simulink model "exp2_latest_work_of_FULL_HEART_PICTURE_orignal_pure"  (R2023a)
settings: Solver=VariableStepAuto  StartTime=0.0  StopTime=60  RelTol=1e-3  AbsTol=1e-3
libraries: fl_lib x40, sh_lib x21, nesl_utility x18, simulink x7, Cardiovascular_lib x4
(part 1 of 2)
settings Model: Creator=luca  LastModifiedBy=Syed Abdul Rahman
settings SolverCC: AutoScaleAbsTol=off  ZeroCrossAlgorithm=Adaptive  AlgebraicLoopSolver=TrustRegion
settings DataIOCC: InspectSignalLogs=on
settings DebuggingCC: IgnoredZcDiagnostic=none  UnconnectedInputMsg=warning  UnconnectedOutputMsg=warning  UnconnectedLineMsg=warning  SymbolicDimsDataTypeCodeGenerationDiagnostic=none
settings ModelReferenceCC: EnableRefExpFcnMdlSchedulingChecks=on
settings SFSimCC: CustomCodeUndefinedFunction=UseInterfaceOnly
settings SimscapeCC: SimscapeLogType=all  SimscapeLogSimulationStatistics=on  SimscapeLogDataHistory=10000

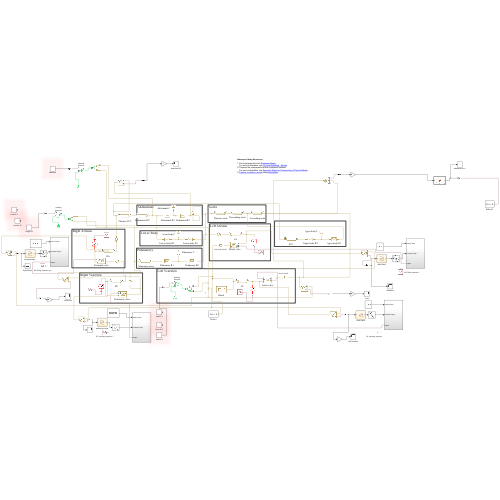
[thumbnail: Simulink's stored preview of the top-level diagram]
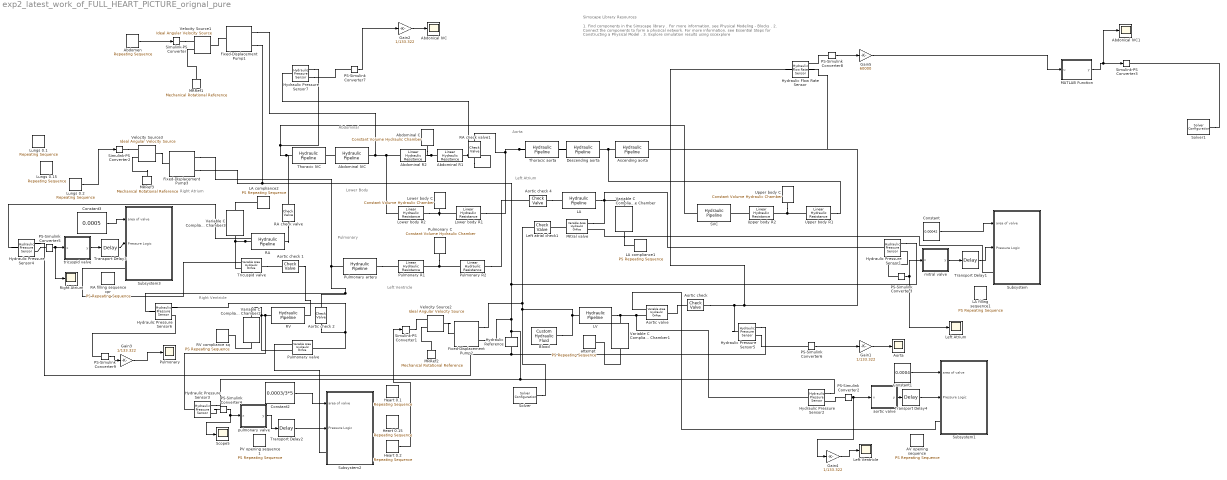
== system exp2_latest_work_of_FULL_HEART_PICTURE_orignal_pure ==
  note: Lower Body
  note: Left Atrium
  note: Right Ventricle
  note: Abdominal
  note: Aorta
  note: 1. Find components in the Simscape library .
      | For more information, see Physical Modeling - Blocks .
      | 2. Connect the components to form a physical network.
      | For more information, see Essential Steps for Constructing a Physical Model .
      | 3. Explore simulation results using sscexplore
  note: Simscape Library Resources
  note: Left Ventricle
  note: Right Atrium
  note: Pulmonary
  AV opening sequence : fl_lib/Physical Signals/Sources/PS Repeating Sequence  y_init=0  offset=0 s  sig_type=2  durations=[0.01 0.01 0.01 0.01 0.01 0.01 0.01 0.01 0.01 0.01 0.01 0.01 0.01 0.01 0.01 0.01 0.01 0.01 0.01 0.01 0.01 0.01 0.01 0.01 0.01 0.01 0.01 0.01 0.01 0.01 0.01 0.01 0.01 0.01 0.01 0.01 0.01 0.01 0.01 0.01 0.01 0.01 0.01 0.01 0.01 0.01 0.01 0.01 0.01 0.01 0.01 0.01 0.01 0.01 0.01 0.01 0.01 0.01 0.01 0.01 0.01 0.01 0.01 0.01 0.01 0.01 0.01 0.01 0.01 0.01 0.01 0.01 0.01 0.01 0.01 0.01 0.01 0.01 0.01 0.01 0.01 0.01 0.01 0.01 0.01 0.01 0.01 0.01 0.01 0.01 0.01 0.01 0.01 0.01 0.01 0.01 0.01 0.01 0.01 0.01] s  y_start="[0.000300000000000000\t0.000300000000000000\t0.000300000000000000\t0.000300000000000000\t0.000300000000000000\t0.000300000000000000\t0.000300000000000000\t0.000300000000000000\t0.000300000000000000\t0.000300000000000000\t0.000300000000000000\t0.000300000000000000\t0.000300000000000000\t0.000300000000000000\t0.000300000000000000\t0.000300000000000000\t0.000300000000000000\t0.000300000000000000\t0.000300000000000000\t0.000300000000000000\t0.000300000000000000\t0.000300000000000000\t0.000300000000000000\t0.000300000000000000\t0.000300000000000000\t0.000300000000000000\t0.000300000000000000\t0.000300000000000000\t0.000300000000000000\t0.000300000000000000\t0.000300000000000000\t0.000300000000000000\t0.000300000000000000\t0.000300000000000000\t0.000300000000000000\t0.000300000000000000\t0.000300000000000000\t0.000300000000000000\t0.000300000000000000\t0.000300000000000000\t0.000300000000000000\t0.000300000000000000\t0.000300000000000000\t0\t0\t0\t0\t0\t0\t0\t0\t0\t0\t0\t0\t0\t0\t0\t0\t0\t0\t0\t0\t0\t0\t0\t0\t0\t0\t0\t0\t0\t0\t0\t0\t0\t0\t0\t0\t0\t0\t0\t0\t0\t0\t0\t0\t0\t0\t0\t0\t0\t0\t0\t0\t0\t0\t0\t0\t0]/3*4"  y_end=1
      settings: InternalSimscapePortConfiguration="{\"Bottom\":[],\"Left\":[],\"Right\":[{\"id\":\"Y\",\"label\":\"Y\",\"type\":\"output\"}],\"Top\":[]}"
  "Abdomen " : simulink/Sources/Repeating Sequence  rep_seq_t=a1  rep_seq_y=a2
  Abdominal C : fl_lib/Hydraulic/Hydraulic Elements/Constant Volume Hydraulic Chamber  ch_sp=2  wall_type=2  ch_volume=1e-4 m^3  d_in=1 cm  length=2570.700637 cm  pr_r_coef=3.6E-08 m/Pa  time_const=0.01 s  k_sh=1.4  pressure_specify=off  pressure_priority=High  pressure=0 Pa  pressure_nominal_specify=off  pressure_nominal_unit=Pa  pressure_nominal_value=1  diameter_incr_specify=off  diameter_incr_priority=High  diameter_incr=0 m  diameter_incr_nominal_specify=off  diameter_incr_nominal_unit=m  diameter_incr_nominal_value=1  flow_rate_specify=off  flow_rate_priority=None  flow_rate=0.001 m^3/s  flow_rate_nominal_specify=off  flow_rate_nominal_unit=m^3/s  flow_rate_nominal_value=1
      settings: InternalSimscapePortConfiguration="{\"Bottom\":[],\"Left\":[{\"id\":\"A\",\"label\":\"\",\"type\":\"foundation.hydraulic.hydraulic\"}],\"Right\":[],\"Top\":[]}"
  Abdominal IVC : sh_lib/Pipelines/Hydraulic Pipeline  cs_type=1  d_in=1.37 cm  area=1e-4 m^2  D_h=1.12e-2 m  s_factor=64  length=17 cm  length_ad=0 m  roughness=15e-6 m  Re_lam=2000  Re_turb=4000  wall_type=2  pr_r_coef=4.39e-6 m/Pa  time_const=0.01 s  k_sh=1.4  initial_pressure=0 Pa
      settings: InternalSimscapePortConfiguration="{\"Bottom\":[],\"Left\":[{\"id\":\"A\",\"label\":\"A\",\"type\":\"foundation.hydraulic.hydraulic\"}],\"Right\":[{\"id\":\"B\",\"label\":\"B\",\"type\":\"foundation.hydraulic.hydraulic\"}],\"Top\":[]}"
  Abdominal R1 : fl_lib/Hydraulic/Hydraulic Elements/Linear Hydraulic Resistance  resistance=2.3e8 Pa/(m^3/s)  q_specify=off  q_priority=None  q=0.001 m^3/s  q_nominal_specify=off  q_nominal_unit=m^3/s  q_nominal_value=1  p_specify=off  p_priority=None  p=0 Pa  p_nominal_specify=off  p_nominal_unit=Pa  p_nominal_value=1
      settings: InternalSimscapePortConfiguration="{\"Bottom\":[],\"Left\":[{\"id\":\"A\",\"label\":\"A\",\"type\":\"foundation.hydraulic.hydraulic\"}],\"Right\":[{\"id\":\"B\",\"label\":\"B\",\"type\":\"foundation.hydraulic.hydraulic\"}],\"Top\":[]}"
  Abdominal R2 : fl_lib/Hydraulic/Hydraulic Elements/Linear Hydraulic Resistance  resistance=0.15e8 Pa/(m^3/s)  q_specify=off  q_priority=None  q=0.001 m^3/s  q_nominal_specify=off  q_nominal_unit=m^3/s  q_nominal_value=1  p_specify=off  p_priority=None  p=0 Pa  p_nominal_specify=off  p_nominal_unit=Pa  p_nominal_value=1
      settings: InternalSimscapePortConfiguration="{\"Bottom\":[],\"Left\":[{\"id\":\"A\",\"label\":\"A\",\"type\":\"foundation.hydraulic.hydraulic\"}],\"Right\":[{\"id\":\"B\",\"label\":\"B\",\"type\":\"foundation.hydraulic.hydraulic\"}],\"Top\":[]}"
  Abdonical IVC : Scope
  Abdonical IVC1 : Scope
  Aorta : Scope
  "Aortic check " : sh_lib/Valves/Directional Valves/Check Valve  area_max=1e-1 m^2  pres_crack=0.01 Pa  pres_max=0.1 Pa  C_d=1  A_leak=1e-12 m^2  lam_spec=1  B_lam=0.999  Re_cr=12  dynamic=0  tau=0.1 s  area_init=1e-12 m^2
      settings: InternalSimscapePortConfiguration="{\"Bottom\":[],\"Left\":[{\"id\":\"A\",\"label\":\"A\",\"type\":\"foundation.hydraulic.hydraulic\"}],\"Right\":[{\"id\":\"B\",\"label\":\"B\",\"type\":\"foundation.hydraulic.hydraulic\"}],\"Top\":[]}"
  Aortic check 1 : sh_lib/Valves/Directional Valves/Check Valve  area_max=1e-1 m^2  pres_crack=0.01 Pa  pres_max=0.1 Pa  C_d=1  A_leak=1e-12 m^2  lam_spec=1  B_lam=0.999  Re_cr=12  dynamic=0  tau=0.1 s  area_init=1e-12 m^2
      settings: InternalSimscapePortConfiguration="{\"Bottom\":[],\"Left\":[{\"id\":\"A\",\"label\":\"A\",\"type\":\"foundation.hydraulic.hydraulic\"}],\"Right\":[{\"id\":\"B\",\"label\":\"B\",\"type\":\"foundation.hydraulic.hydraulic\"}],\"Top\":[]}"
  Aortic check 2 : sh_lib/Valves/Directional Valves/Check Valve  area_max=1e-1 m^2  pres_crack=0.01 Pa  pres_max=0.1 Pa  C_d=1  A_leak=1e-12 m^2  lam_spec=1  B_lam=0.999  Re_cr=12  dynamic=0  tau=0.1 s  area_init=1e-12 m^2
      settings: InternalSimscapePortConfiguration="{\"Bottom\":[],\"Left\":[{\"id\":\"A\",\"label\":\"A\",\"type\":\"foundation.hydraulic.hydraulic\"}],\"Right\":[{\"id\":\"B\",\"label\":\"B\",\"type\":\"foundation.hydraulic.hydraulic\"}],\"Top\":[]}"
  Aortic check 4 : sh_lib/Valves/Directional Valves/Check Valve  area_max=1e-3 m^2  pres_crack=0.01 Pa  pres_max=0.1 Pa  C_d=1  A_leak=1e-12 m^2  lam_spec=1  B_lam=0.999  Re_cr=12  dynamic=0  tau=0.1 s  area_init=1e-12 m^2
      settings: InternalSimscapePortConfiguration="{\"Bottom\":[],\"Left\":[{\"id\":\"A\",\"label\":\"A\",\"type\":\"foundation.hydraulic.hydraulic\"}],\"Right\":[{\"id\":\"B\",\"label\":\"B\",\"type\":\"foundation.hydraulic.hydraulic\"}],\"Top\":[]}"
  Aortic valve : fl_lib/Hydraulic/Hydraulic Elements/Variable Area Hydraulic Orifice  C_d=1  min_area=1e-15 m^2  lam_spec=1  B_lam=0.999  Re_cr=12  q_specify=off  q_priority=None  q=0.001 m^3/s  q_nominal_specify=off  q_nominal_unit=m^3/s  q_nominal_value=1  p_specify=off  p_priority=None  p=0 Pa  p_nominal_specify=off  p_nominal_unit=Pa  p_nominal_value=1
      settings: InternalSimscapePortConfiguration="{\"Bottom\":[],\"Left\":[{\"id\":\"AR\",\"label\":\"AR\",\"type\":\"input\"},{\"id\":\"A\",\"label\":\"A\",\"type\":\"foundation.hydraulic.hydraulic\"}],\"Right\":[{\"id\":\"B\",\"label\":\"B\",\"type\":\"foundation.hydraulic.hydraulic\"}],\"Top\":[]}"
  Ascending aorta : sh_lib/Pipelines/Hydraulic Pipeline  cs_type=1  d_in=2.65 cm  area=1e-4 m^2  D_h=1.12e-2 m  s_factor=64  length=8.8 cm  length_ad=0 m  roughness=15e-6 m  Re_lam=2000  Re_turb=4000  wall_type=2  pr_r_coef=4.5e-7 m/Pa  time_const=0.01 s  k_sh=1.4  initial_pressure=0 Pa
      settings: InternalSimscapePortConfiguration="{\"Bottom\":[],\"Left\":[{\"id\":\"A\",\"label\":\"A\",\"type\":\"foundation.hydraulic.hydraulic\"}],\"Right\":[{\"id\":\"B\",\"label\":\"B\",\"type\":\"foundation.hydraulic.hydraulic\"}],\"Top\":[]}"
  "Blood " : fl_lib/Hydraulic/Hydraulic Utilities/Custom Hydraulic Fluid  density=1060 kg/m^3  viscosity_kin=3.55e-6 m^2/s  bulk=2.2e9 Pa  alpha=0.005  range_error=2
      settings: InternalSimscapePortConfiguration="{\"Bottom\":[],\"Left\":[],\"Right\":[{\"id\":\"G\",\"label\":\"\",\"type\":\"foundation.hydraulic.hydraulic\"}],\"Top\":[]}"
  Constant : Constant  Value=0.00042
  Constant1 : Constant  Value=0.0004
  Constant2 : Constant  Value=0.0003/3*5
  Constant3 : Constant  Value=0.0005
  Descending aorta : sh_lib/Pipelines/Hydraulic Pipeline  cs_type=1  d_in=2.15 cm  area=1e-4 m^2  D_h=1.12e-2 m  s_factor=64  length=6.94 cm  length_ad=0 m  roughness=15e-6 m  Re_lam=2000  Re_turb=4000  wall_type=2  pr_r_coef=1.4e-6 m/Pa  time_const=0.01 s  k_sh=1.4  initial_pressure=0 Pa
      settings: InternalSimscapePortConfiguration="{\"Bottom\":[],\"Left\":[{\"id\":\"A\",\"label\":\"A\",\"type\":\"foundation.hydraulic.hydraulic\"}],\"Right\":[{\"id\":\"B\",\"label\":\"B\",\"type\":\"foundation.hydraulic.hydraulic\"}],\"Top\":[]}"
  Fixed-Displacement Pump1 : sh_lib/Pumps and Motors/Fixed-Displacement Pump  D=13.33 cm^3/rev  loss_spec=1  w_nominal=20 rpm  pr_nominal=100e5 Pa  visc_nominal=3.55e-6 m^2/s  dens_nominal=1060 kg/m^3  efficiency_vol=0.92  no_load_torque=0.05 N*m  torque_pressure_coeff=0.6e-6 N*m/Pa  p_diff_eff_TLU=[100000, 1000000, 2000000] Pa  omega_eff_TLU=[25, 50, 100, 200, 300, 400] rad/s  vol_eff_TLU=[.816, .908, .954, .977, .981, .984; .325, .663, .831, .916, .925, .946; .137, .568, .78, .892, .893, .91]  mech_eff_TLU=[.996, .996, .996, .996, .996, .996; .988, .989, .989, .989, .989, .99; .981, .981, .982, .982, .983, .984]  p_diff_loss_TLU=[100000, 1000000, 2000000] Pa  omega_loss_TLU=[25, 50, 100, 200, 300, 400] rad/s  vol_loss_TLU=[.023, .023, .023, .023, .0285, .032; .0844, .0842, .0845, .084, .1125, .108; .1079, .108, .11, .108, .1605, .18] * 1e-3 m^3/s  mech_loss_TLU=[.002, .002, .002, .002, .002, .002; .0607, .0556, .0556, .0556, .0556, .0505; .1937, .1937, .1833, .1833, .1729, .1626] N*m  pressure_threshold=1e5 Pa  omega_threshold=10 rad/s  quadrant_check=0  pressure_check=0  min_valid_pressure=0 Pa  vol_eff_min=1e-3  vol_eff_max=1  mech_eff_min=1e-3  mech_eff_max=1
      settings: InternalSimscapePortConfiguration="{\"Bottom\":[],\"Left\":[{\"id\":\"S\",\"label\":\"S\",\"type\":\"foundation.mechanical.rotational.rotational\"}],\"Right\":[{\"id\":\"P\",\"label\":\"P\",\"type\":\"foundation.hydraulic.hydraulic\"},{\"id\":\"T\",\"label\":\"T\",\"type\":\"foundation.hydraulic.hydraulic\"}],\"Top\":[]}"
  Fixed-Displacement Pump2 : sh_lib/Pumps and Motors/Fixed-Displacement Pump  D=13.33 cm^3/rev  loss_spec=1  w_nominal=20 rpm  pr_nominal=100e5 Pa  visc_nominal=3.55e-6 m^2/s  dens_nominal=1060 kg/m^3  efficiency_vol=0.92  no_load_torque=0.05 N*m  torque_pressure_coeff=0.6e-6 N*m/Pa  p_diff_eff_TLU=[100000, 1000000, 2000000] Pa  omega_eff_TLU=[25, 50, 100, 200, 300, 400] rad/s  vol_eff_TLU=[.816, .908, .954, .977, .981, .984; .325, .663, .831, .916, .925, .946; .137, .568, .78, .892, .893, .91]  mech_eff_TLU=[.996, .996, .996, .996, .996, .996; .988, .989, .989, .989, .989, .99; .981, .981, .982, .982, .983, .984]  p_diff_loss_TLU=[100000, 1000000, 2000000] Pa  omega_loss_TLU=[25, 50, 100, 200, 300, 400] rad/s  vol_loss_TLU=[.023, .023, .023, .023, .0285, .032; .0844, .0842, .0845, .084, .1125, .108; .1079, .108, .11, .108, .1605, .18] * 1e-3 m^3/s  mech_loss_TLU=[.002, .002, .002, .002, .002, .002; .0607, .0556, .0556, .0556, .0556, .0505; .1937, .1937, .1833, .1833, .1729, .1626] N*m  pressure_threshold=1e5 Pa  omega_threshold=10 rad/s  quadrant_check=0  pressure_check=0  min_valid_pressure=0 Pa  vol_eff_min=1e-3  vol_eff_max=1  mech_eff_min=1e-3  mech_eff_max=1
      settings: InternalSimscapePortConfiguration="{\"Bottom\":[],\"Left\":[{\"id\":\"S\",\"label\":\"S\",\"type\":\"foundation.mechanical.rotational.rotational\"}],\"Right\":[{\"id\":\"P\",\"label\":\"P\",\"type\":\"foundation.hydraulic.hydraulic\"},{\"id\":\"T\",\"label\":\"T\",\"type\":\"foundation.hydraulic.hydraulic\"}],\"Top\":[]}"
  Fixed-Displacement Pump3 : sh_lib/Pumps and Motors/Fixed-Displacement Pump  D=13.33 cm^3/rev  loss_spec=1  w_nominal=20 rpm  pr_nominal=100e5 Pa  visc_nominal=3.55e-6 m^2/s  dens_nominal=1060 kg/m^3  efficiency_vol=0.92  no_load_torque=0.05 N*m  torque_pressure_coeff=0.6e-6 N*m/Pa  p_diff_eff_TLU=[100000, 1000000, 2000000] Pa  omega_eff_TLU=[25, 50, 100, 200, 300, 400] rad/s  vol_eff_TLU=[.816, .908, .954, .977, .981, .984; .325, .663, .831, .916, .925, .946; .137, .568, .78, .892, .893, .91]  mech_eff_TLU=[.996, .996, .996, .996, .996, .996; .988, .989, .989, .989, .989, .99; .981, .981, .982, .982, .983, .984]  p_diff_loss_TLU=[100000, 1000000, 2000000] Pa  omega_loss_TLU=[25, 50, 100, 200, 300, 400] rad/s  vol_loss_TLU=[.023, .023, .023, .023, .0285, .032; .0844, .0842, .0845, .084, .1125, .108; .1079, .108, .11, .108, .1605, .18] * 1e-3 m^3/s  mech_loss_TLU=[.002, .002, .002, .002, .002, .002; .0607, .0556, .0556, .0556, .0556, .0505; .1937, .1937, .1833, .1833, .1729, .1626] N*m  pressure_threshold=1e5 Pa  omega_threshold=10 rad/s  quadrant_check=0  pressure_check=0  min_valid_pressure=0 Pa  vol_eff_min=1e-3  vol_eff_max=1  mech_eff_min=1e-3  mech_eff_max=1
      settings: InternalSimscapePortConfiguration="{\"Bottom\":[],\"Left\":[{\"id\":\"S\",\"label\":\"S\",\"type\":\"foundation.mechanical.rotational.rotational\"}],\"Right\":[{\"id\":\"P\",\"label\":\"P\",\"type\":\"foundation.hydraulic.hydraulic\"},{\"id\":\"T\",\"label\":\"T\",\"type\":\"foundation.hydraulic.hydraulic\"}],\"Top\":[]}"
  Gain{1..4} (4 alike) : Gain  Gain=1/133.322
  Gain5 : Gain  Gain=60000
  Heart 0.1 : simulink/Sources/Repeating Sequence  rep_seq_t=b1  rep_seq_y=b2
  Heart 0.15 : simulink/Sources/Repeating Sequence  rep_seq_t=c1  rep_seq_y=c2
  Heart 0.2 : simulink/Sources/Repeating Sequence  rep_seq_t=d1  rep_seq_y=d2
  Hydraulic Flow Rate Sensor : fl_lib/Hydraulic/Hydraulic Sensors/Hydraulic Flow Rate Sensor
  Hydraulic Pressure Sensor{1..7} (7 alike) : fl_lib/Hydraulic/Hydraulic Sensors/Hydraulic Pressure Sensor
  Hydraulic Reference : fl_lib/Hydraulic/Hydraulic Elements/Hydraulic Reference
  LA : sh_lib/Pipelines/Hydraulic Pipeline  cs_type=1  d_in=4.8 cm  area=1e-4 m^2  D_h=1.12e-2 m  s_factor=64  length=5 cm  length_ad=0 m  roughness=15e-6 m  Re_lam=2000  Re_turb=4000  wall_type=1  pr_r_coef=5.9e-6 m/Pa  time_const=0.01 s  k_sh=1.4  initial_pressure=0 Pa
      settings: InternalSimscapePortConfiguration="{\"Bottom\":[],\"Left\":[{\"id\":\"A\",\"label\":\"A\",\"type\":\"foundation.hydraulic.hydraulic\"}],\"Right\":[{\"id\":\"B\",\"label\":\"B\",\"type\":\"foundation.hydraulic.hydraulic\"}],\"Top\":[]}"
  LA compliance1 : fl_lib/Physical Signals/Sources/PS Repeating Sequence  y_init=0  offset=0 s  sig_type=2  durations=[0.01 0.01 0.01 0.01 0.01 0.01 0.01 0.01 0.01 0.01 0.01 0.01 0.01 0.01 0.01 0.01 0.01 0.01 0.01 0.01 0.01 0.01 0.01 0.01 0.01 0.01 0.01 0.01 0.01 0.01 0.01 0.01 0.01 0.01 0.01 0.01 0.01 0.01 0.01 0.01 0.01 0.01 0.01 0.01 0.01 0.01 0.01 0.01 0.01 0.01 0.01 0.01 0.01 0.01 0.01 0.01 0.01 0.01 0.01 0.01 0.01 0.01 0.01 0.01 0.01 0.01 0.01 0.01 0.01 0.01 0.01 0.01 0.01 0.01 0.01 0.01 0.01 0.01 0.01 0.01 0.01 0.01 0.01 0.01 0.01 0.01 0.01 0.01 0.01 0.01 0.01 0.01 0.01 0.01 0.01 0.01 0.01 0.01 0.01 0.01] s  y_start="[1.36500000000000e-05\t1.36862500000000e-05\t1.37225000000000e-05\t1.37587500000000e-05\t1.37950000000000e-05\t1.38312500000000e-05\t1.38675000000000e-05\t1.39037500000000e-05\t1.39400000000000e-05\t1.39762500000000e-05\t1.40125000000000e-05\t1.40487500000000e-05\t1.40850000000000e-05\t1.41212500000000e-05\t1.41575000000000e-05\t1.41937500000000e-05\t1.42300000000000e-05\t1.42662500000000e-05\t1.43025000000000e-05\t1.43387500000000e-05\t1.43750000000000e-05\t1.44112500000000e-05\t1.44475000000000e-05\t1.44837500000000e-05\t1.45200000000000e-05\t1.45562500000000e-05\t1.45925000000000e-05\t1.46287500000000e-05\t1.46650000000000e-05\t1.47012500000000e-05\t1.47375000000000e-05\t1.47737500000000e-05\t1.48100000000000e-05\t1.48462500000000e-05\t1.48825000000000e-05\t1.49187500000000e-05\t1.49550000000000e-05\t1.49912500000000e-05\t1.50275000000000e-05\t1.50637500000000e-05\t1.51000000000000e-05\t1.51362500000000e-05\t1.51725000000000e-05\t1.52087500000000e-05\t1.52450000000000e-05\t1.52812500000000e-05\t1.53175000000000e-05\t1.53537500000000e-05\t1.53900000000000e-05\t1.54262500000000e-05\t1.54625000000000e-05\t1.54987500000000e-05\t1.55350000000000e-05\t1.55712500000000e-05\t1.56075000000000e-05\t1.56437500000000e-05\t1.56800000000000e-05\t1.57162500000000e-05\t1.57525000000000e-05\t1.57887500000000e-05\t1.58250000000000e-05\t1.58612500000000e-05\t1.58975000000000e-05\t1.59337500000000e-05\t1.59700000000000e-05\t1.60062500000000e-05\t1.60425000000000e-05\t1.60787500000000e-05\t1.61150000000000e-05\t1.61512500000000e-05\t1.61875000000000e-05\t1.62237500000000e-05\t1.62600000000000e-05\t1.62962500000000e-05\t1.63325000000000e-05\t1.63687500000000e-05\t1.64050000000000e-05\t1.64412500000000e-05\t1.64775000000000e-05\t1.65137500000000e-05\t1.36500000000000e-05\t1.29125270139567e-05\t1.21876723951708e-05\t1.14878386071372e-05\t1.08250000000000e-05\t1.02104979261007e-05\t9.65484668629601e-06\t9.16755362735452e-06\t8.75695646861792e-06\t8.43008064131123e-06\t8.19251908146676e-06\t8.04833653323797e-06\t8.00000000000000e-06\t8.14165729617270e-06\t8.55952589635133e-06\t9.23265212405563e-06\t1.01272826194982e-05\t1.11985568739858e-05\t1.23927567231468e-05\t1.36500000000000e-05]"  y_end=1
      settings: InternalSimscapePortConfiguration="{\"Bottom\":[],\"Left\":[],\"Right\":[{\"id\":\"Y\",\"label\":\"Y\",\"type\":\"output\"}],\"Top\":[]}"
  LA compliance2 : fl_lib/Physical Signals/Sources/PS Repeating Sequence  y_init=0  offset=0 s  sig_type=2  durations=[0.01 0.01 0.01 0.01 0.01 0.01 0.01 0.01 0.01 0.01 0.01 0.01 0.01 0.01 0.01 0.01 0.01 0.01 0.01 0.01 0.01 0.01 0.01 0.01 0.01 0.01 0.01 0.01 0.01 0.01 0.01 0.01 0.01 0.01 0.01 0.01 0.01 0.01 0.01 0.01 0.01 0.01 0.01 0.01 0.01 0.01 0.01 0.01 0.01 0.01 0.01 0.01 0.01 0.01 0.01 0.01 0.01 0.01 0.01 0.01 0.01 0.01 0.01 0.01 0.01 0.01 0.01 0.01 0.01 0.01 0.01 0.01 0.01 0.01 0.01 0.01 0.01 0.01 0.01 0.01 0.01 0.01 0.01 0.01 0.01 0.01 0.01 0.01 0.01 0.01 0.01 0.01 0.01 0.01 0.01 0.01 0.01 0.01 0.01 0.01] s  y_start="[2.18400000000000e-05\t2.18580000000000e-05\t2.18760000000000e-05\t2.18940000000000e-05\t2.19120000000000e-05\t2.19300000000000e-05\t2.19480000000000e-05\t2.19660000000000e-05\t2.19840000000000e-05\t2.20020000000000e-05\t2.20200000000000e-05\t2.20380000000000e-05\t2.20560000000000e-05\t2.20740000000000e-05\t2.20920000000000e-05\t2.21100000000000e-05\t2.21280000000000e-05\t2.21460000000000e-05\t2.21640000000000e-05\t2.21820000000000e-05\t2.22000000000000e-05\t2.22180000000000e-05\t2.22360000000000e-05\t2.22540000000000e-05\t2.22720000000000e-05\t2.22900000000000e-05\t2.23080000000000e-05\t2.23260000000000e-05\t2.23440000000000e-05\t2.23620000000000e-05\t2.23800000000000e-05\t2.23980000000000e-05\t2.24160000000000e-05\t2.24340000000000e-05\t2.24520000000000e-05\t2.24700000000000e-05\t2.24880000000000e-05\t2.25060000000000e-05\t2.25240000000000e-05\t2.25420000000000e-05\t2.25600000000000e-05\t2.25780000000000e-05\t2.25960000000000e-05\t2.26140000000000e-05\t2.26320000000000e-05\t2.26500000000000e-05\t2.26680000000000e-05\t2.26860000000000e-05\t2.27040000000000e-05\t2.27220000000000e-05\t2.27400000000000e-05\t2.27580000000000e-05\t2.27760000000000e-05\t2.27940000000000e-05\t2.28120000000000e-05\t2.28300000000000e-05\t2.28480000000000e-05\t2.28660000000000e-05\t2.28840000000000e-05\t2.29020000000000e-05\t2.29200000000000e-05\t2.29380000000000e-05\t2.29560000000000e-05\t2.29740000000000e-05\t2.29920000000000e-05\t2.30100000000000e-05\t2.30280000000000e-05\t2.30460000000000e-05\t2.30640000000000e-05\t2.30820000000000e-05\t2.31000000000000e-05\t2.31180000000000e-05\t2.31360000000000e-05\t2.31540000000000e-05\t2.31720000000000e-05\t2.31900000000000e-05\t2.32080000000000e-05\t2.32260000000000e-05\t2.32440000000000e-05\t2.32620000000000e-05\t2.18400000000000e-05\t2.14693056140951e-05\t2.11049539119088e-05\t2.07531790520831e-05\t2.04200000000000e-05\t2.01111175416152e-05\t1.98318167414302e-05\t1.95868765135729e-05\t1.93804878532522e-05\t1.92161821276679e-05\t1.90967706533390e-05\t1.90242965936984e-05\t1.90000000000000e-05\t1.90712047294036e-05\t1.92812484151571e-05\t1.96195985897908e-05\t2.00692889627212e-05\t2.06077701809061e-05\t2.12080405475641e-05\t2.18400000000000e-05]"  y_end=1
      settings: InternalSimscapePortConfiguration="{\"Bottom\":[],\"Left\":[],\"Right\":[{\"id\":\"Y\",\"label\":\"Y\",\"type\":\"output\"}],\"Top\":[]}"
  LA filling sequence1 : fl_lib/Physical Signals/Sources/PS Repeating Sequence  y_init=0  offset=0 s  sig_type=2  durations=[0.01 0.01 0.01 0.01 0.01 0.01 0.01 0.01 0.01 0.01 0.01 0.01 0.01 0.01 0.01 0.01 0.01 0.01 0.01 0.01 0.01 0.01 0.01 0.01 0.01 0.01 0.01 0.01 0.01 0.01 0.01 0.01 0.01 0.01 0.01 0.01 0.01 0.01 0.01 0.01 0.01 0.01 0.01 0.01 0.01 0.01 0.01 0.01 0.01 0.01 0.01 0.01 0.01 0.01 0.01 0.01 0.01 0.01 0.01 0.01 0.01 0.01 0.01 0.01 0.01 0.01 0.01 0.01 0.01 0.01 0.01 0.01 0.01 0.01 0.01 0.01 0.01 0.01 0.01 0.01 0.01 0.01 0.01 0.01 0.01 0.01 0.01 0.01 0.01 0.01 0.01 0.01 0.01 0.01 0.01 0.01 0.01 0.01 0.01 0.01] s  y_start="[0\t0\t0\t0\t0\t0\t0\t0\t0\t0\t0\t0\t0\t0\t0\t0\t0\t0\t0\t0\t0\t0\t0\t0\t0\t0\t0\t0\t0\t0\t0\t0\t0\t0\t0\t0\t0\t0\t0\t0\t0\t0\t0\t0\t0\t0.000420000000000000\t0.000420000000000000\t0.000420000000000000\t0.000420000000000000\t0.000420000000000000\t0.000420000000000000\t0.000420000000000000\t0.000420000000000000\t0.000420000000000000\t0.000420000000000000\t0.000420000000000000\t0.000420000000000000\t0.000420000000000000\t0.000420000000000000\t0.000420000000000000\t0.000420000000000000\t0.000420000000000000\t0.000420000000000000\t0.000420000000000000\t0.000420000000000000\t0.000420000000000000\t0.000420000000000000\t0.000420000000000000\t0.000420000000000000\t0.000420000000000000\t0.000420000000000000\t0.000420000000000000\t0.000420000000000000\t0.000420000000000000\t0.000420000000000000\t0.000420000000000000\t0.000420000000000000\t0.000420000000000000\t0.000420000000000000\t0.000420000000000000\t0.000420000000000000\t0.000420000000000000\t0.000420000000000000\t0.000420000000000000\t0.000420000000000000\t0.000420000000000000\t0.000420000000000000\t0.000420000000000000\t0.000420000000000000\t0.000420000000000000\t0.000420000000000000\t0.000420000000000000\t0.000420000000000000\t0.000420000000000000\t0.000420000000000000\t0.000420000000000000\t0.000420000000000000\t0.000420000000000000\t0.000420000000000000\t0.000420000000000000]"  y_end=1
      settings: InternalSimscapePortConfiguration="{\"Bottom\":[],\"Left\":[],\"Right\":[{\"id\":\"Y\",\"label\":\"Y\",\"type\":\"output\"}],\"Top\":[]}"
  LV : sh_lib/Pipelines/Hydraulic Pipeline  cs_type=1  d_in=4.4 cm  area=1e-4 m^2  D_h=1.12e-2 m  s_factor=64  length=7 cm  length_ad=0 m  roughness=15e-6 m  Re_lam=2000  Re_turb=4000  wall_type=1  pr_r_coef=3.8e-7 m/Pa  time_const=0.01 s  k_sh=1.4  initial_pressure=0 Pa
      settings: InternalSimscapePortConfiguration="{\"Bottom\":[],\"Left\":[{\"id\":\"A\",\"label\":\"A\",\"type\":\"foundation.hydraulic.hydraulic\"}],\"Right\":[{\"id\":\"B\",\"label\":\"B\",\"type\":\"foundation.hydraulic.hydraulic\"}],\"Top\":[]}"
  "Left Atrium " : Scope
  Left Ventricle : Scope
  Left atrial check1 : sh_lib/Valves/Directional Valves/Check Valve  area_max=1e-1 m^2  pres_crack=0.01 Pa  pres_max=0.1 Pa  C_d=0.7  A_leak=1e-12 m^2  lam_spec=1  B_lam=0.999  Re_cr=12  dynamic=0  tau=0.1 s  area_init=1e-12 m^2
      settings: InternalSimscapePortConfiguration="{\"Bottom\":[],\"Left\":[{\"id\":\"A\",\"label\":\"A\",\"type\":\"foundation.hydraulic.hydraulic\"}],\"Right\":[{\"id\":\"B\",\"label\":\"B\",\"type\":\"foundation.hydraulic.hydraulic\"}],\"Top\":[]}"
  Lower body C : fl_lib/Hydraulic/Hydraulic Elements/Constant Volume Hydraulic Chamber  ch_sp=2  wall_type=2  ch_volume=1e-4 m^3  d_in=1 cm  length=648.4076433 cm  pr_r_coef=4.1E-08 m/Pa  time_const=0.01 s  k_sh=1.4  pressure_specify=off  pressure_priority=High  pressure=0 Pa  pressure_nominal_specify=off  pressure_nominal_unit=Pa  pressure_nominal_value=1  diameter_incr_specify=off  diameter_incr_priority=High  diameter_incr=0 m  diameter_incr_nominal_specify=off  diameter_incr_nominal_unit=m  diameter_incr_nominal_value=1  flow_rate_specify=off  flow_rate_priority=None  flow_rate=0.001 m^3/s  flow_rate_nominal_specify=off  flow_rate_nominal_unit=m^3/s  flow_rate_nominal_value=1
      settings: InternalSimscapePortConfiguration="{\"Bottom\":[],\"Left\":[{\"id\":\"A\",\"label\":\"\",\"type\":\"foundation.hydraulic.hydraulic\"}],\"Right\":[],\"Top\":[]}"
  Lower body R1 : fl_lib/Hydraulic/Hydraulic Elements/Linear Hydraulic Resistance  resistance=4.79e8 Pa/(m^3/s)  q_specify=off  q_priority=None  q=0.001 m^3/s  q_nominal_specify=off  q_nominal_unit=m^3/s  q_nominal_value=1  p_specify=off  p_priority=None  p=0 Pa  p_nominal_specify=off  p_nominal_unit=Pa  p_nominal_value=1
      settings: InternalSimscapePortConfiguration="{\"Bottom\":[],\"Left\":[{\"id\":\"A\",\"label\":\"A\",\"type\":\"foundation.hydraulic.hydraulic\"}],\"Right\":[{\"id\":\"B\",\"label\":\"B\",\"type\":\"foundation.hydraulic.hydraulic\"}],\"Top\":[]}"
  Lower body R2 : fl_lib/Hydraulic/Hydraulic Elements/Linear Hydraulic Resistance  resistance=0.4e8 Pa/(m^3/s)  q_specify=off  q_priority=None  q=0.001 m^3/s  q_nominal_specify=off  q_nominal_unit=m^3/s  q_nominal_value=1  p_specify=off  p_priority=None  p=0 Pa  p_nominal_specify=off  p_nominal_unit=Pa  p_nominal_value=1
      settings: InternalSimscapePortConfiguration="{\"Bottom\":[],\"Left\":[{\"id\":\"A\",\"label\":\"A\",\"type\":\"foundation.hydraulic.hydraulic\"}],\"Right\":[{\"id\":\"B\",\"label\":\"B\",\"type\":\"foundation.hydraulic.hydraulic\"}],\"Top\":[]}"
  Lungs 0.1 : simulink/Sources/Repeating Sequence  rep_seq_t=m1  rep_seq_y=m2
  Lungs 0.15 : simulink/Sources/Repeating Sequence  rep_seq_t=n1  rep_seq_y=n2
  Lungs 0.2 : simulink/Sources/Repeating Sequence  rep_seq_t=o1  rep_seq_y=o2
  MATLAB Function : MATLAB Function  TreatAsAtomicUnit=on
  MRRef1 : fl_lib/Mechanical/Rotational Elements/Mechanical Rotational Reference  Tag=Factory Generic
  MRRef2 : fl_lib/Mechanical/Rotational Elements/Mechanical Rotational Reference  Tag=Factory Generic
  MRRef3 : fl_lib/Mechanical/Rotational Elements/Mechanical Rotational Reference  Tag=Factory Generic
  Mitral valve : fl_lib/Hydraulic/Hydraulic Elements/Variable Area Hydraulic Orifice  C_d=1  min_area=1e-15 m^2  lam_spec=1  B_lam=0.999  Re_cr=12  q_specify=off  q_priority=None  q=0.001 m^3/s  q_nominal_specify=off  q_nominal_unit=m^3/s  q_nominal_value=1  p_specify=off  p_priority=None  p=0 Pa  p_nominal_specify=off  p_nominal_unit=Pa  p_nominal_value=1
      settings: InternalSimscapePortConfiguration="{\"Bottom\":[],\"Left\":[{\"id\":\"AR\",\"label\":\"AR\",\"type\":\"input\"},{\"id\":\"A\",\"label\":\"A\",\"type\":\"foundation.hydraulic.hydraulic\"}],\"Right\":[{\"id\":\"B\",\"label\":\"B\",\"type\":\"foundation.hydraulic.hydraulic\"}],\"Top\":[]}"
  PS-Simulink Converter{2..9} (8 alike) : nesl_utility/PS-Simulink Converter  PhysicalDomain=network_engine_domain  SubClassName=ps_output  LeftPortType=input  RightPortType=output  PseudoPeriodic=off  Frequencies=[]  VectorFormat=1-D array  Unit=inherit  AffineConversion=off
  PV opening sequence 1 : fl_lib/Physical Signals/Sources/PS Repeating Sequence  y_init=0  offset=0 s  sig_type=2  durations=[0.01 0.01 0.01 0.01 0.01 0.01 0.01 0.01 0.01 0.01 0.01 0.01 0.01 0.01 0.01 0.01 0.01 0.01 0.01 0.01 0.01 0.01 0.01 0.01 0.01 0.01 0.01 0.01 0.01 0.01 0.01 0.01 0.01 0.01 0.01 0.01 0.01 0.01 0.01 0.01 0.01 0.01 0.01 0.01 0.01 0.01 0.01 0.01 0.01 0.01 0.01 0.01 0.01 0.01 0.01 0.01 0.01 0.01 0.01 0.01 0.01 0.01 0.01 0.01 0.01 0.01 0.01 0.01 0.01 0.01 0.01 0.01 0.01 0.01 0.01 0.01 0.01 0.01 0.01 0.01 0.01 0.01 0.01 0.01 0.01 0.01 0.01 0.01 0.01 0.01 0.01 0.01 0.01 0.01 0.01 0.01 0.01 0.01 0.01 0.01] s  y_start="[0.000300000000000000\t0.000300000000000000\t0.000300000000000000\t0.000300000000000000\t0.000300000000000000\t0.000300000000000000\t0.000300000000000000\t0.000300000000000000\t0.000300000000000000\t0.000300000000000000\t0.000300000000000000\t0.000300000000000000\t0.000300000000000000\t0.000300000000000000\t0.000300000000000000\t0.000300000000000000\t0.000300000000000000\t0.000300000000000000\t0.000300000000000000\t0.000300000000000000\t0.000300000000000000\t0.000300000000000000\t0.000300000000000000\t0.000300000000000000\t0.000300000000000000\t0.000300000000000000\t0.000300000000000000\t0.000300000000000000\t0.000300000000000000\t0.000300000000000000\t0.000300000000000000\t0.000300000000000000\t0.000300000000000000\t0.000300000000000000\t0.000300000000000000\t0.000300000000000000\t0.000300000000000000\t0.000300000000000000\t0.000300000000000000\t0.000300000000000000\t0.000300000000000000\t0.000300000000000000\t0.000300000000000000\t0.000300000000000000\t0.000300000000000000\t\t0.000300000000000000\t0.000300000000000000\t0.000300000000000000\t0.000300000000000000\t0.000300000000000000\t0.000300000000000000\t0.000300000000000000\t0.000300000000000000\t0\t0\t0\t0\t0\t0\t0\t0\t0\t0\t0\t0\t0\t0\t0\t0\t0\t0\t0\t0\t0\t0\t0\t0\t0\t0\t0\t0\t0\t0\t0\t0\t0\t0\t0\t0\t0\t0\t0\t0\t0\t0\t0 0 0 0 0]/3*5"  y_end=1
      settings: InternalSimscapePortConfiguration="{\"Bottom\":[],\"Left\":[],\"Right\":[{\"id\":\"Y\",\"label\":\"Y\",\"type\":\"output\"}],\"Top\":[]}"
  Pulmonary : Scope
  Pulmonary C : fl_lib/Hydraulic/Hydraulic Elements/Constant Volume Hydraulic Chamber  ch_sp=2  wall_type=2  ch_volume=1e-4 m^3  d_in=1 cm  length=702.4 cm  pr_r_coef=6e-7 m/Pa  time_const=0.01 s  k_sh=1.4  pressure_specify=off  pressure_priority=High  pressure=0 Pa  pressure_nominal_specify=off  pressure_nominal_unit=Pa  pressure_nominal_value=1  diameter_incr_specify=off  diameter_incr_priority=High  diameter_incr=0 m  diameter_incr_nominal_specify=off  diameter_incr_nominal_unit=m  diameter_incr_nominal_value=1  flow_rate_specify=off  flow_rate_priority=None  flow_rate=0.001 m^3/s  flow_rate_nominal_specify=off  flow_rate_nominal_unit=m^3/s  flow_rate_nominal_value=1
      settings: InternalSimscapePortConfiguration="{\"Bottom\":[],\"Left\":[{\"id\":\"A\",\"label\":\"\",\"type\":\"foundation.hydraulic.hydraulic\"}],\"Right\":[],\"Top\":[]}"
  Pulmonary R1 : fl_lib/Hydraulic/Hydraulic Elements/Linear Hydraulic Resistance  resistance=0.5e7 Pa/(m^3/s)  q_specify=off  q_priority=None  q=0.001 m^3/s  q_nominal_specify=off  q_nominal_unit=m^3/s  q_nominal_value=1  p_specify=off  p_priority=None  p=0 Pa  p_nominal_specify=off  p_nominal_unit=Pa  p_nominal_value=1
      settings: InternalSimscapePortConfiguration="{\"Bottom\":[],\"Left\":[{\"id\":\"A\",\"label\":\"A\",\"type\":\"foundation.hydraulic.hydraulic\"}],\"Right\":[{\"id\":\"B\",\"label\":\"B\",\"type\":\"foundation.hydraulic.hydraulic\"}],\"Top\":[]}"
  Pulmonary R2 : fl_lib/Hydraulic/Hydraulic Elements/Linear Hydraulic Resistance  resistance=0.05e7 Pa/(m^3/s)  q_specify=off  q_priority=None  q=0.001 m^3/s  q_nominal_specify=off  q_nominal_unit=m^3/s  q_nominal_value=1  p_specify=off  p_priority=None  p=0 Pa  p_nominal_specify=off  p_nominal_unit=Pa  p_nominal_value=1
      settings: InternalSimscapePortConfiguration="{\"Bottom\":[],\"Left\":[{\"id\":\"A\",\"label\":\"A\",\"type\":\"foundation.hydraulic.hydraulic\"}],\"Right\":[{\"id\":\"B\",\"label\":\"B\",\"type\":\"foundation.hydraulic.hydraulic\"}],\"Top\":[]}"
  Pulmonary artery : sh_lib/Pipelines/Hydraulic Pipeline  cs_type=1  d_in=3 cm  area=1e-4 m^2  D_h=1.12e-2 m  s_factor=64  length=5 cm  length_ad=0 m  roughness=15e-6 m  Re_lam=2000  Re_turb=4000  wall_type=2  pr_r_coef=2.2e-7 m/Pa  time_const=0.01 s  k_sh=1.4  initial_pressure=0 Pa
      settings: InternalSimscapePortConfiguration="{\"Bottom\":[],\"Left\":[{\"id\":\"A\",\"label\":\"A\",\"type\":\"foundation.hydraulic.hydraulic\"}],\"Right\":[{\"id\":\"B\",\"label\":\"B\",\"type\":\"foundation.hydraulic.hydraulic\"}],\"Top\":[]}"
  Pulmonary valve : fl_lib/Hydraulic/Hydraulic Elements/Variable Area Hydraulic Orifice  C_d=1  min_area=1e-15 m^2  lam_spec=1  B_lam=0.999  Re_cr=12  q_specify=off  q_priority=None  q=0.001 m^3/s  q_nominal_specify=off  q_nominal_unit=m^3/s  q_nominal_value=1  p_specify=off  p_priority=None  p=0 Pa  p_nominal_specify=off  p_nominal_unit=Pa  p_nominal_value=1
      settings: InternalSimscapePortConfiguration="{\"Bottom\":[],\"Left\":[{\"id\":\"AR\",\"label\":\"AR\",\"type\":\"input\"},{\"id\":\"A\",\"label\":\"A\",\"type\":\"foundation.hydraulic.hydraulic\"}],\"Right\":[{\"id\":\"B\",\"label\":\"B\",\"type\":\"foundation.hydraulic.hydraulic\"}],\"Top\":[]}"
  RA : sh_lib/Pipelines/Hydraulic Pipeline  cs_type=1  d_in=5.6 cm  area=1e-4 m^2  D_h=1.12e-2 m  s_factor=64  length=5 cm  length_ad=0 m  roughness=15e-6 m  Re_lam=2000  Re_turb=4000  wall_type=1  pr_r_coef=5.9e-6 m/Pa  time_const=0.01 s  k_sh=1.4  initial_pressure=0 Pa
      settings: InternalSimscapePortConfiguration="{\"Bottom\":[],\"Left\":[{\"id\":\"A\",\"label\":\"A\",\"type\":\"foundation.hydraulic.hydraulic\"}],\"Right\":[{\"id\":\"B\",\"label\":\"B\",\"type\":\"foundation.hydraulic.hydraulic\"}],\"Top\":[]}"
  RA check valve : sh_lib/Valves/Directional Valves/Check Valve  area_max=1e-1 m^2  pres_crack=0.01 Pa  pres_max=0.1 Pa  C_d=1  A_leak=1e-12 m^2  lam_spec=1  B_lam=0.999  Re_cr=12  dynamic=0  tau=0.1 s  area_init=1e-12 m^2
      settings: InternalSimscapePortConfiguration="{\"Bottom\":[],\"Left\":[{\"id\":\"A\",\"label\":\"A\",\"type\":\"foundation.hydraulic.hydraulic\"}],\"Right\":[{\"id\":\"B\",\"label\":\"B\",\"type\":\"foundation.hydraulic.hydraulic\"}],\"Top\":[]}"
  RA check valve1 : sh_lib/Valves/Directional Valves/Check Valve  area_max=1e-1 m^2  pres_crack=0.01 Pa  pres_max=0.1 Pa  C_d=1  A_leak=1e-12 m^2  lam_spec=1  B_lam=0.999  Re_cr=12  dynamic=0  tau=0.1 s  area_init=1e-12 m^2
      settings: InternalSimscapePortConfiguration="{\"Bottom\":[],\"Left\":[{\"id\":\"A\",\"label\":\"A\",\"type\":\"foundation.hydraulic.hydraulic\"}],\"Right\":[{\"id\":\"B\",\"label\":\"B\",\"type\":\"foundation.hydraulic.hydraulic\"}],\"Top\":[]}"
  RA filling sequence cpr : fl_lib/Physical Signals/Sources/PS Repeating Sequence  y_init=0  offset=0 s  sig_type=2  durations=[0.01 0.01 0.01 0.01 0.01 0.01 0.01 0.01 0.01 0.01 0.01 0.01 0.01 0.01 0.01 0.01 0.01 0.01 0.01 0.01 0.01 0.01 0.01 0.01 0.01 0.01 0.01 0.01 0.01 0.01 0.01 0.01 0.01 0.01 0.01 0.01 0.01 0.01 0.01 0.01 0.01 0.01 0.01 0.01 0.01 0.01 0.01 0.01 0.01 0.01 0.01 0.01 0.01 0.01 0.01 0.01 0.01 0.01 0.01 0.01 0.01 0.01 0.01 0.01 0.01 0.01 0.01 0.01 0.01 0.01 0.01 0.01 0.01 0.01 0.01 0.01 0.01 0.01 0.01 0.01 0.01 0.01 0.01 0.01 0.01 0.01 0.01 0.01 0.01 0.01 0.01 0.01 0.01 0.01 0.01 0.01 0.01 0.01 0.01 0.01] s  y_start="[0\t0\t0\t0\t0\t0\t0\t0\t0\t0\t0\t0\t0\t0\t0\t0\t0\t0\t0\t0\t0\t0\t0\t0\t0\t0\t0\t0\t0\t0\t0\t0\t0\t0\t0\t0\t0\t0\t0\t0\t0\t0\t0\t0\t0\t0.000500000000000000\t0.000500000000000000\t0.000500000000000000\t0.000500000000000000\t0.000500000000000000\t0.000500000000000000\t0.000500000000000000\t0.000500000000000000\t0.000500000000000000\t0.000500000000000000\t0.000500000000000000\t0.000500000000000000\t0.000500000000000000\t0.000500000000000000\t0.000500000000000000\t0.000500000000000000\t0.000500000000000000\t0.000500000000000000\t0.000500000000000000\t0.000500000000000000\t0.000500000000000000\t0.000500000000000000\t0.000500000000000000\t0.000500000000000000\t0.000500000000000000\t0.000500000000000000\t0.000500000000000000\t0.000500000000000000\t0.000500000000000000\t0.000500000000000000\t0.000500000000000000\t0.000500000000000000\t0.000500000000000000\t0.000500000000000000\t0.000500000000000000\t0.000500000000000000\t0.000500000000000000\t0.000500000000000000\t0.000500000000000000\t0.000500000000000000\t0.000500000000000000\t0.000500000000000000\t0.000500000000000000\t0.000500000000000000\t0.000500000000000000\t0.000500000000000000\t0.000500000000000000\t0.000500000000000000\t0.000500000000000000\t0.000500000000000000\t0.000500000000000000\t0.000500000000000000\t0.000500000000000000\t0.000500000000000000\t0.000500000000000000]"  y_end=1
      settings: InternalSimscapePortConfiguration="{\"Bottom\":[],\"Left\":[],\"Right\":[{\"id\":\"Y\",\"label\":\"Y\",\"type\":\"output\"}],\"Top\":[]}"
  RV : sh_lib/Pipelines/Hydraulic Pipeline  cs_type=1  d_in=5 cm  area=1e-4 m^2  D_h=1.12e-2 m  s_factor=64  length=7.5 cm  length_ad=0 m  roughness=15e-6 m  Re_lam=2000  Re_turb=4000  wall_type=1  pr_r_coef=3.8e-7 m/Pa  time_const=0.01 s  k_sh=1.4  initial_pressure=0 Pa
      settings: InternalSimscapePortConfiguration="{\"Bottom\":[],\"Left\":[{\"id\":\"A\",\"label\":\"A\",\"type\":\"foundation.hydraulic.hydraulic\"}],\"Right\":[{\"id\":\"B\",\"label\":\"B\",\"type\":\"foundation.hydraulic.hydraulic\"}],\"Top\":[]}"
  RV compliance sq : fl_lib/Physical Signals/Sources/PS Repeating Sequence  y_init=0  offset=0 s  sig_type=2  durations=[0.01 0.01 0.01 0.01 0.01 0.01 0.01 0.01 0.01 0.01 0.01 0.01 0.01 0.01 0.01 0.01 0.01 0.01 0.01 0.01 0.01 0.01 0.01 0.01 0.01 0.01 0.01 0.01 0.01 0.01 0.01 0.01 0.01 0.01 0.01 0.01 0.01 0.01 0.01 0.01 0.01 0.01 0.01 0.01 0.01 0.01 0.01 0.01 0.01 0.01 0.01 0.01 0.01 0.01 0.01 0.01 0.01 0.01 0.01 0.01 0.01 0.01 0.01 0.01 0.01 0.01 0.01 0.01 0.01 0.01 0.01 0.01 0.01 0.01 0.01 0.01 0.01 0.01 0.01 0.01 0.01 0.01 0.01 0.01 0.01 0.01 0.01 0.01 0.01 0.01 0.01 0.01 0.01 0.01 0.01 0.01 0.01 0.01 0.01 0.01] s  y_start="[5.50000000000000e-05\t5.26294018607136e-05\t5.02685450176733e-05\t4.79271307380492e-05\t4.56147803953482e-05\t4.33409959331260e-05\t4.11151208194632e-05\t3.89463016526504e-05\t3.68434505758543e-05\t3.48152086552097e-05\t3.28699103718250e-05\t3.10155493736118e-05\t2.92597456276710e-05\t2.76097141082133e-05\t2.60722351486829e-05\t2.46536265799126e-05\t2.33597177688022e-05\t2.21958256641990e-05\t2.11667329484149e-05\t2.02766683841589e-05\t1.95292894376436e-05\t1.89276672492725e-05\t1.84742740136653e-05\t1.81709728208797e-05\t1.80190100005745e-05\t1.80190100005745e-05\t1.81709728208797e-05\t1.84742740136653e-05\t1.89276672492725e-05\t1.95292894376436e-05\t2.02766683841589e-05\t2.11667329484149e-05\t2.21958256641990e-05\t2.33597177688022e-05\t2.46536265799126e-05\t2.60722351486829e-05\t2.76097141082133e-05\t2.92597456276710e-05\t3.10155493736118e-05\t3.28699103718250e-05\t3.48152086552097e-05\t3.68434505758543e-05\t3.89463016526503e-05\t4.11151208194631e-05\t4.33409959331260e-05\t4.56147803953482e-05\t4.79271307380492e-05\t5.02685450176733e-05\t5.26294018607136e-05\t5.50000000000000e-05\t5.50000000000000e-05\t5.50000000000000e-05\t5.50000000000000e-05\t5.50000000000000e-05\t5.50000000000000e-05\t5.50000000000000e-05\t5.50000000000000e-05\t5.50000000000000e-05\t5.50000000000000e-05\t5.50000000000000e-05\t5.50000000000000e-05\t5.50000000000000e-05\t5.50000000000000e-05\t5.50000000000000e-05\t5.50000000000000e-05\t5.50000000000000e-05\t5.50000000000000e-05\t5.50000000000000e-05\t5.50000000000000e-05\t5.50000000000000e-05\t5.50000000000000e-05\t5.50000000000000e-05\t5.50000000000000e-05\t5.50000000000000e-05\t5.50000000000000e-05\t5.50000000000000e-05\t5.50000000000000e-05\t5.50000000000000e-05\t5.50000000000000e-05\t5.50000000000000e-05\t5.50000000000000e-05\t5.50000000000000e-05\t5.50000000000000e-05\t5.50000000000000e-05\t5.50000000000000e-05\t5.50000000000000e-05\t5.50000000000000e-05\t5.50000000000000e-05\t5.50000000000000e-05\t5.50000000000000e-05\t5.50000000000000e-05\t5.50000000000000e-05\t5.50000000000000e-05\t5.50000000000000e-05\t5.50000000000000e-05\t5.50000000000000e-05\t5.50000000000000e-05\t5.50000000000000e-05\t5.50000000000000e-05\t5.50000000000000e-05]"  y_end=1
      settings: InternalSimscapePortConfiguration="{\"Bottom\":[],\"Left\":[],\"Right\":[{\"id\":\"Y\",\"label\":\"Y\",\"type\":\"output\"}],\"Top\":[]}"
  Right Atrium : Scope
  SVC : sh_lib/Pipelines/Hydraulic Pipeline  cs_type=1  d_in=2.1 cm  area=1e-4 m^2  D_h=1.12e-2 m  s_factor=64  length=7.1 cm  length_ad=0 m  roughness=15e-6 m  Re_lam=2000  Re_turb=4000  wall_type=2  pr_r_coef=5e-6 m/Pa  time_const=0.01 s  k_sh=1.4  initial_pressure=0 Pa
      settings: InternalSimscapePortConfiguration="{\"Bottom\":[],\"Left\":[{\"id\":\"A\",\"label\":\"A\",\"type\":\"foundation.hydraulic.hydraulic\"}],\"Right\":[{\"id\":\"B\",\"label\":\"B\",\"type\":\"foundation.hydraulic.hydraulic\"}],\"Top\":[]}"
  Scope5 : Scope
  Simulink-PS Converter{,1..3} (4 alike) : nesl_utility/Simulink-PS Converter  PhysicalDomain=network_engine_domain  SubClassName=ps_input  LeftPortType=input  RightPortType=output  PseudoPeriodic=off  Frequencies=[]  NoiseDistribution=none  NoiseParameters=[]  Unit=1  AffineConversion=off  FilteringAndDerivatives=provide  SimscapeFilterOrder=1  InputFilterTimeConstant=0.001  UdotUserProvided=0
  Solver : nesl_utility/Solver Configuration  PhysicalDomain=network_engine_domain  SubClassName=solver  LeftPortType=input  RightPortType=generic  Tones=[]  Harmonics=[]  SimulateNoise=off  Profile=off  UseLocalSampling=off  EnableSwitchedLinearOptims=on  FrequencyDomain=off  UseCCode=off  RelTol=0.001  AbsTol=1e-06  MinStep=1e-09  ToWorkspace=off  RevertToSquareIcSolve=off  NumHomotopyIterations=100  PhasorMode=off  PhasorModeNumHarmonics=1  ConsistencySolver=NEWTON_FTOL  IndexReductionMethod=DerivativeReplacement  DoDC=off  ResidualTolerance=1e-09  ConsistencyTolSource=GLOBAL  ConsistencyAbsTol=0.001  ConsistencyRelTol=0.001  ConsistencyTolFactor=0.001  UseLocalSolver=off  LocalSolverChoice=NE_BACKWARD_EULER_ADVANCER  ResolveIndetEquations=on  FunctionEvalNumThread=1  LocalSolverSampleTime=0.001  DoFixedCost=off  MaxNonlinIter=3  MaxModeIter=2  ComputeImpulses=off  ImpulseIterations=2  LinearAlgebra=auto  LinearAlgebraNumThread=0  EquationFormulation=NE_TIME_EF  DelaysMemoryBudget=1024  AutomaticFiltering=on  FilteringTimeConstant=0.00001  PartitionStorageMethod=AS_NEEDED  PartitionMemoryBudget=1024  PartitionMethod=ROBUST
  Solver1 : nesl_utility/Solver Configuration  PhysicalDomain=network_engine_domain  SubClassName=solver  LeftPortType=input  RightPortType=generic  Tones=[]  Harmonics=[]  SimulateNoise=off  Profile=off  UseLocalSampling=off  EnableSwitchedLinearOptims=on  FrequencyDomain=off  UseCCode=off  RelTol=0.001  AbsTol=1e-06  MinStep=1e-09  ToWorkspace=off  RevertToSquareIcSolve=off  NumHomotopyIterations=100  PhasorMode=off  PhasorModeNumHarmonics=1  ConsistencySolver=NEWTON_FTOL  IndexReductionMethod=DerivativeReplacement  DoDC=off  ResidualTolerance=1e-09  ConsistencyTolSource=GLOBAL  ConsistencyAbsTol=0.001  ConsistencyRelTol=0.001  ConsistencyTolFactor=0.001  UseLocalSolver=off  LocalSolverChoice=NE_BACKWARD_EULER_ADVANCER  ResolveIndetEquations=on  FunctionEvalNumThread=1  LocalSolverSampleTime=0.001  DoFixedCost=off  MaxNonlinIter=3  MaxModeIter=2  ComputeImpulses=off  ImpulseIterations=2  LinearAlgebra=auto  LinearAlgebraNumThread=0  EquationFormulation=NE_TIME_EF  DelaysMemoryBudget=1024  AutomaticFiltering=on  FilteringTimeConstant=0.00001  PartitionStorageMethod=AS_NEEDED  PartitionMemoryBudget=1024  PartitionMethod=ROBUST
  Subsystem : Subsystem
  Subsystem1 : Subsystem
  Subsystem2 : Subsystem
  Subsystem3 : Subsystem
  Thoracic IVC : sh_lib/Pipelines/Hydraulic Pipeline  cs_type=1  d_in=1.37 cm  area=1e-4 m^2  D_h=1.12e-2 m  s_factor=64  length=2.5 cm  length_ad=0 m  roughness=15e-6 m  Re_lam=2000  Re_turb=4000  wall_type=2  pr_r_coef=6.37e-7 m/Pa  time_const=0.01 s  k_sh=1.4  initial_pressure=0 Pa
      settings: InternalSimscapePortConfiguration="{\"Bottom\":[],\"Left\":[{\"id\":\"A\",\"label\":\"A\",\"type\":\"foundation.hydraulic.hydraulic\"}],\"Right\":[{\"id\":\"B\",\"label\":\"B\",\"type\":\"foundation.hydraulic.hydraulic\"}],\"Top\":[]}"
  Thoracic aorta : sh_lib/Pipelines/Hydraulic Pipeline  cs_type=1  d_in=1.92 cm  area=1e-4 m^2  D_h=1.12e-2 m  s_factor=64  length=33.2 cm  length_ad=0 m  roughness=15e-6 m  Re_lam=2000  Re_turb=4000  wall_type=2  pr_r_coef=3.3e-7 m/Pa  time_const=0.01 s  k_sh=1.4  initial_pressure=0 Pa
      settings: InternalSimscapePortConfiguration="{\"Bottom\":[],\"Left\":[{\"id\":\"A\",\"label\":\"A\",\"type\":\"foundation.hydraulic.hydraulic\"}],\"Right\":[{\"id\":\"B\",\"label\":\"B\",\"type\":\"foundation.hydraulic.hydraulic\"}],\"Top\":[]}"
  Transport Delay{1..4} (4 alike) : TransportDelay  DelayTime=0.001  BufferSize=30720
  Tricuspid valve : fl_lib/Hydraulic/Hydraulic Elements/Variable Area Hydraulic Orifice  C_d=1  min_area=1e-15 m^2  lam_spec=1  B_lam=0.999  Re_cr=12  q_specify=off  q_priority=None  q=0.001 m^3/s  q_nominal_specify=off  q_nominal_unit=m^3/s  q_nominal_value=1  p_specify=off  p_priority=None  p=0 Pa  p_nominal_specify=off  p_nominal_unit=Pa  p_nominal_value=1
      settings: InternalSimscapePortConfiguration="{\"Bottom\":[],\"Left\":[{\"id\":\"AR\",\"label\":\"AR\",\"type\":\"input\"},{\"id\":\"A\",\"label\":\"A\",\"type\":\"foundation.hydraulic.hydraulic\"}],\"Right\":[{\"id\":\"B\",\"label\":\"B\",\"type\":\"foundation.hydraulic.hydraulic\"}],\"Top\":[]}"
  Upper body C : fl_lib/Hydraulic/Hydraulic Elements/Constant Volume Hydraulic Chamber  ch_sp=2  wall_type=2  ch_volume=1e-4 m^3  d_in=1 cm  length=1131.210191 cm  pr_r_coef=6.7E-08 m/Pa  time_const=0.01 s  k_sh=1.4  pressure_specify=off  pressure_priority=High  pressure=0 Pa  pressure_nominal_specify=off  pressure_nominal_unit=Pa  pressure_nominal_value=1  diameter_incr_specify=off  diameter_incr_priority=High  diameter_incr=0 m  diameter_incr_nominal_specify=off  diameter_incr_nominal_unit=m  diameter_incr_nominal_value=1  flow_rate_specify=off  flow_rate_priority=None  flow_rate=0.001 m^3/s  flow_rate_nominal_specify=off  flow_rate_nominal_unit=m^3/s  flow_rate_nominal_value=1
      settings: InternalSimscapePortConfiguration="{\"Bottom\":[],\"Left\":[{\"id\":\"A\",\"label\":\"\",\"type\":\"foundation.hydraulic.hydraulic\"}],\"Right\":[],\"Top\":[]}"
  Upper body R1 : fl_lib/Hydraulic/Hydraulic Elements/Linear Hydraulic Resistance  resistance=5.19e8 Pa/(m^3/s)  q_specify=off  q_priority=None  q=0.001 m^3/s  q_nominal_specify=off  q_nominal_unit=m^3/s  q_nominal_value=1  p_specify=off  p_priority=None  p=0 Pa  p_nominal_specify=off  p_nominal_unit=Pa  p_nominal_value=1
      settings: InternalSimscapePortConfiguration="{\"Bottom\":[],\"Left\":[{\"id\":\"A\",\"label\":\"A\",\"type\":\"foundation.hydraulic.hydraulic\"}],\"Right\":[{\"id\":\"B\",\"label\":\"B\",\"type\":\"foundation.hydraulic.hydraulic\"}],\"Top\":[]}"
  Upper body R2 : fl_lib/Hydraulic/Hydraulic Elements/Linear Hydraulic Resistance  resistance=0.31e8 Pa/(m^3/s)  q_specify=off  q_priority=None  q=0.001 m^3/s  q_nominal_specify=off  q_nominal_unit=m^3/s  q_nominal_value=1  p_specify=off  p_priority=None  p=0 Pa  p_nominal_specify=off  p_nominal_unit=Pa  p_nominal_value=1
      settings: InternalSimscapePortConfiguration="{\"Bottom\":[],\"Left\":[{\"id\":\"A\",\"label\":\"A\",\"type\":\"foundation.hydraulic.hydraulic\"}],\"Right\":[{\"id\":\"B\",\"label\":\"B\",\"type\":\"foundation.hydraulic.hydraulic\"}],\"Top\":[]}"
  Variable C Compliance Chamber{,1..3} (4 alike) : Cardiovascular_lib/Variable C Compliance Chamber  d_in=1e-2 m  length=1 m  time_const=0.01 s  k_sh=1.4  pressure_specify=off  pressure_priority=High  pressure=0 Pa  pressure_nominal_specify=off  pressure_nominal_unit=Pa  pressure_nominal_value=1  diameter_incr_specify=off  diameter_incr_priority=High  diameter_incr=0 m  diameter_incr_nominal_specify=off  diameter_incr_nominal_unit=m  diameter_incr_nominal_value=1  flow_rate_specify=off  flow_rate_priority=None  flow_rate=1e-3 m^3/s  flow_rate_nominal_specify=off  flow_rate_nominal_unit=m^3/s  flow_rate_nominal_value=1
      settings: InternalSimscapePortConfiguration="{\"Bottom\":[],\"Left\":[{\"id\":\"A\",\"label\":\"\",\"type\":\"foundation.hydraulic.hydraulic\"}],\"Right\":[{\"id\":\"V\",\"label\":\"C\",\"type\":\"input\"}],\"Top\":[]}"
  Velocity Source1 : fl_lib/Mechanical/Mechanical Sources/Ideal Angular Velocity Source  Tag=Factory Generic
  Velocity Source2 : fl_lib/Mechanical/Mechanical Sources/Ideal Angular Velocity Source  Tag=Factory Generic
  Velocity Source3 : fl_lib/Mechanical/Mechanical Sources/Ideal Angular Velocity Source  Tag=Factory Generic
  aortic valve : Stateflow chart  TreatAsAtomicUnit=on
  attempt : fl_lib/Physical Signals/Sources/PS Repeating Sequence  y_init=0  offset=0 s  sig_type=2  durations=[0.01 0.01 0.01 0.01 0.01 0.01 0.01 0.01 0.01 0.01 0.01 0.01 0.01 0.01 0.01 0.01 0.01 0.01 0.01 0.01 0.01 0.01 0.01 0.01 0.01 0.01 0.01 0.01 0.01 0.01 0.01 0.01 0.01 0.01 0.01 0.01 0.01 0.01 0.01 0.01 0.01 0.01 0.01 0.01 0.01 0.01 0.01 0.01 0.01 0.01 0.01 0.01 0.01 0.01 0.01 0.01 0.01 0.01 0.01 0.01 0.01 0.01 0.01 0.01 0.01 0.01 0.01 0.01 0.01 0.01 0.01 0.01 0.01 0.01 0.01] s  y_start="[1.00000000000000e-06\t9.37357264520457e-07\t8.74971941477825e-07\t8.13100385546094e-07\t7.51996840219996e-07\t6.91912393073946e-07\t6.33093943989338e-07\t5.75783190589981e-07\t5.20215635054710e-07\t4.66619616388422e-07\t4.15215372128128e-07\t3.66214133339669e-07\t3.19817256623959e-07\t2.76215396699523e-07\t2.35587722961358e-07\t1.98101183235464e-07\t1.63909817754413e-07\t1.33154126172990e-07\t1.05960490224980e-07\t8.24406543935084e-08\t6.26912667289963e-08\t4.67934817015874e-08\t3.48126267200239e-08\t2.67979336873100e-08\t2.27823366962635e-08\t2.27823366962635e-08\t2.67979336873100e-08\t3.48126267200239e-08\t4.67934817015874e-08\t6.26912667289962e-08\t8.24406543935083e-08\t1.05960490224980e-07\t1.33154126172990e-07\t1.63909817754413e-07\t1.98101183235464e-07\t2.35587722961358e-07\t2.76215396699523e-07\t3.19817256623959e-07\t3.66214133339669e-07\t4.15215372128128e-07\t4.66619616388422e-07\t5.20215635054710e-07\t5.75783190589981e-07\t6.33093943989338e-07\t6.91912393073945e-07\t7.51996840219996e-07\t8.13100385546094e-07\t8.74971941477825e-07\t9.37357264520457e-07\t1.00000000000000e-06\t1.00000000000000e-06\t1.00000000000000e-06\t1.00000000000000e-06\t1.00000000000000e-06\t1.00000000000000e-06\t1.50000000000000e-06\t1.50000000000000e-06\t1.50000000000000e-06\t1.50000000000000e-06\t1.50000000000000e-06\t1.50000000000000e-06\t1.50000000000000e-06\t1.50000000000000e-06\t1.50000000000000e-06\t1.50000000000000e-06\t1.50000000000000e-06\t1.50000000000000e-06\t1.50000000000000e-06\t1.50000000000000e-06\t1.50000000000000e-06\t1.50000000000000e-06\t1.50000000000000e-06\t1.50000000000000e-06\t1.50000000000000e-06\t1.50000000000000e-06]"  y_end=1
      settings: InternalSimscapePortConfiguration="{\"Bottom\":[],\"Left\":[],\"Right\":[{\"id\":\"Y\",\"label\":\"Y\",\"type\":\"output\"}],\"Top\":[]}"
  mitral valve : Stateflow chart  TreatAsAtomicUnit=on
  pulmonary valve : Stateflow chart  TreatAsAtomicUnit=on
  "tricuspid valve " : Stateflow chart  TreatAsAtomicUnit=on
  wires:
  Constant/1 -> Subsystem/1(area of valve)
  PS-Simulink Converter3/1 -> "Left Atrium "/1, mitral valve/1(x)
  Transport Delay1/1 -> Subsystem/2("Pressure Logic ")
  mitral valve/1(y) -> Transport Delay1/1
  Constant1/1 -> Subsystem1/1(area of valve)
  Transport Delay4/1 -> Subsystem1/2("Pressure Logic ")
  aortic valve/1(y) -> Transport Delay4/1
  PS-Simulink Converter2/1 -> Gain4/1, aortic valve/1(x)
  Constant2/1 -> Subsystem2/1(area of valve)
  pulmonary valve/1(y) -> Transport Delay2/1
  Transport Delay2/1 -> Subsystem2/2("Pressure Logic ")
  PS-Simulink Converter4/1 -> Scope5/1, pulmonary valve/1(x)
  "tricuspid valve "/1(y) -> Transport Delay3/1
  Transport Delay3/1 -> Subsystem3/2("Pressure Logic ")
  Constant3/1 -> Subsystem3/1(area of valve)
  PS-Simulink Converter5/1 -> Right Atrium/1, "tricuspid valve "/1(x)
  PS-Simulink Converter7/1 -> Gain2/1
  "Abdomen "/1 -> Simulink-PS Converter/1
  PS-Simulink Converter9/1 -> Gain3/1
  Gain3/1 -> Pulmonary/1
  PS-Simulink Converter6/1 -> Gain1/1
  Gain1/1 -> Aorta/1
  Gain5/1 -> MATLAB Function/1(u)
  MATLAB Function/1(y) -> Abdonical IVC1/1, Simulink-PS Converter3/1
  PS-Simulink Converter8/1 -> Gain5/1
  Gain2/1 -> Abdonical IVC/1
  Gain4/1 -> Left Ventricle/1
  Lungs 0.2/1 -> Simulink-PS Converter2/1
  Heart 0.2/1 -> Simulink-PS Converter1/1
  connections:
  Hydraulic Reference/LConn1 -- Hydraulic Pressure Sensor2/RConn1 -- Hydraulic Pressure Sensor3/RConn1 -- Hydraulic Pressure Sensor4/RConn1 -- Hydraulic Pressure Sensor5/RConn1 -- Fixed-Displacement Pump3/RConn2 -- Fixed-Displacement Pump1/RConn2 -- Hydraulic Pressure Sensor1/RConn1 -- Fixed-Displacement Pump2/RConn2
  Subsystem3/LConn1 -- Tricuspid valve/LConn1
  LV/RConn1 -- Variable C Compliance Chamber1/LConn1 -- Hydraulic Pressure Sensor2/LConn1 -- Aortic valve/LConn2
  Upper body R1/RConn1 -- Upper body C/LConn1 -- Upper body R2/LConn1
  Pulmonary R2/LConn1 -- Pulmonary C/LConn1 -- Pulmonary R1/RConn1
  Variable C Compliance Chamber3/RConn1 -- LA compliance2/RConn1
  Abdominal R1/RConn1 -- Abdominal C/LConn1 -- Abdominal R2/LConn1
  Lower body R2/LConn1 -- Lower body C/LConn1 -- Lower body R1/RConn1
  Pulmonary artery/RConn1 -- Pulmonary R1/LConn1
  Lower body R1/LConn1 -- Hydraulic Flow Rate Sensor/RConn2 -- Thoracic aorta/RConn1 -- RA check valve1/LConn1
  Ascending aorta/RConn1 -- Upper body R1/LConn1 -- Descending aorta/LConn1
  Thoracic aorta/LConn1 -- Descending aorta/RConn1
  Upper body R2/RConn1 -- SVC/LConn1
  Abdominal R2/RConn1 -- Lower body R2/RConn1 -- Fixed-Displacement Pump1/RConn1 -- Abdominal IVC/LConn1
  Abdominal IVC/RConn1 -- Thoracic IVC/LConn1
  Pulmonary R2/RConn1 -- Aortic check 4/LConn1
  Variable C Compliance Chamber2/RConn1 -- RV compliance sq/RConn1
  RV/RConn1 -- Hydraulic Pressure Sensor3/LConn1 -- Variable C Compliance Chamber2/LConn1 -- Pulmonary valve/LConn2
  RA/RConn1 -- Hydraulic Pressure Sensor4/LConn1 -- Variable C Compliance Chamber3/LConn1 -- Tricuspid valve/LConn2
  Mitral valve/LConn2 -- Variable C Compliance Chamber/LConn1 -- Hydraulic Pressure Sensor1/LConn1 -- LA/RConn1
  Pulmonary artery/LConn1 -- Fixed-Displacement Pump3/RConn1 -- Aortic check 2/RConn1 -- Hydraulic Pressure Sensor6/LConn1
  RA check valve/RConn1 -- RA/LConn1
  Tricuspid valve/RConn1 -- Aortic check 1/LConn1
  Variable C Compliance Chamber/RConn1 -- LA compliance1/RConn1
  Variable C Compliance Chamber1/RConn1 -- attempt/RConn1
  Subsystem1/LConn1 -- Aortic valve/LConn1
  Subsystem/LConn1 -- Mitral valve/LConn1
  Mitral valve/RConn1 -- Left atrial check1/LConn1
  Aortic check 4/RConn1 -- LA/LConn1
  "Aortic check "/LConn1 -- Aortic valve/RConn1
  Aortic check 2/LConn1 -- Hydraulic Pressure Sensor6/RConn1 -- Pulmonary valve/RConn1
  RA check valve/LConn1 -- Hydraulic Pressure Sensor7/RConn1 -- SVC/RConn1 -- Thoracic IVC/RConn1
  Aortic check 1/RConn1 -- RV/LConn1
  "Aortic check "/RConn1 -- Hydraulic Pressure Sensor5/LConn1 -- Hydraulic Flow Rate Sensor/LConn1 -- Ascending aorta/LConn1
  PS-Simulink Converter3/LConn1 -- Hydraulic Pressure Sensor1/RConn2
  PS-Simulink Converter2/LConn1 -- Hydraulic Pressure Sensor2/RConn2
  Pulmonary valve/LConn1 -- Subsystem2/LConn1
  PS-Simulink Converter4/LConn1 -- Hydraulic Pressure Sensor3/RConn2
  PS-Simulink Converter5/LConn1 -- Hydraulic Pressure Sensor4/RConn2
  Fixed-Displacement Pump1/LConn1 -- Velocity Source1/LConn1
  MRRef1/LConn1 -- Velocity Source1/RConn2
  Left atrial check1/RConn1 -- Fixed-Displacement Pump2/RConn1 -- "Blood "/RConn1 -- LV/LConn1 -- Solver/RConn1
  RA check valve1/RConn1 -- Hydraulic Pressure Sensor7/LConn1 -- Abdominal R1/LConn1
  Hydraulic Pressure Sensor5/RConn2 -- PS-Simulink Converter6/LConn1
  MRRef2/LConn1 -- Velocity Source2/RConn2
  Velocity Source2/LConn1 -- Fixed-Displacement Pump2/LConn1
  PS-Simulink Converter9/LConn1 -- Hydraulic Pressure Sensor6/RConn2
  Hydraulic Pressure Sensor7/RConn2 -- PS-Simulink Converter7/LConn1
  Simulink-PS Converter/RConn1 -- Velocity Source1/RConn1
  Simulink-PS Converter1/RConn1 -- Velocity Source2/RConn1
  Simulink-PS Converter2/RConn1 -- Velocity Source3/RConn1
  MRRef3/LConn1 -- Velocity Source3/RConn2
  Velocity Source3/LConn1 -- Fixed-Displacement Pump3/LConn1
  PS-Simulink Converter8/LConn1 -- Hydraulic Flow Rate Sensor/RConn1
  Solver1/RConn1 -- Simulink-PS Converter3/RConn1
